simulink model "MinMax"  (R2023b)
settings: Solver=VariableStepAuto  StartTime=0.0  StopTime=10.0  RelTol=1e-3
settings Model: Creator=hp  LastModifiedBy=hp

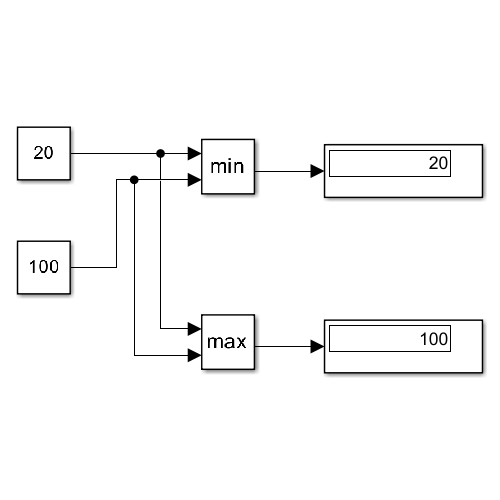
[thumbnail: Simulink's stored preview of the top-level diagram]
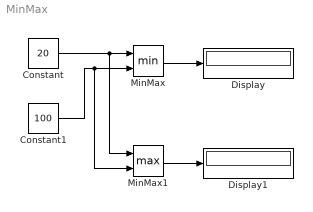
== system MinMax ==
  Constant : Constant  Value=20
  Constant1 : Constant  Value=100
  Display : Display
  Display1 : Display
  MinMax : MinMax  Inputs=2
  MinMax1 : MinMax  Function=max  Inputs=2
  wires:
  Constant/1 -> MinMax1/1, MinMax/1
  Constant1/1 -> MinMax1/2, MinMax/2
  MinMax/1 -> Display/1
  MinMax1/1 -> Display1/1
